simulink model "Robot Michał Krzyszczuk"  (R2018b)
settings: Solver=VariableStepAuto  StartTime=0.0  StopTime=500  MaxStep=0.001  RelTol=1e-3
libraries: commrandsrc3 x9
settings Model: Creator=lenovo  LastModifiedBy=michask
settings SFSimCC: SimUseLocalCustomCode=off
settings RTWCC: RTWUseLocalCustomCode=off
settings CodeAppCC: StateflowObjectComments=on

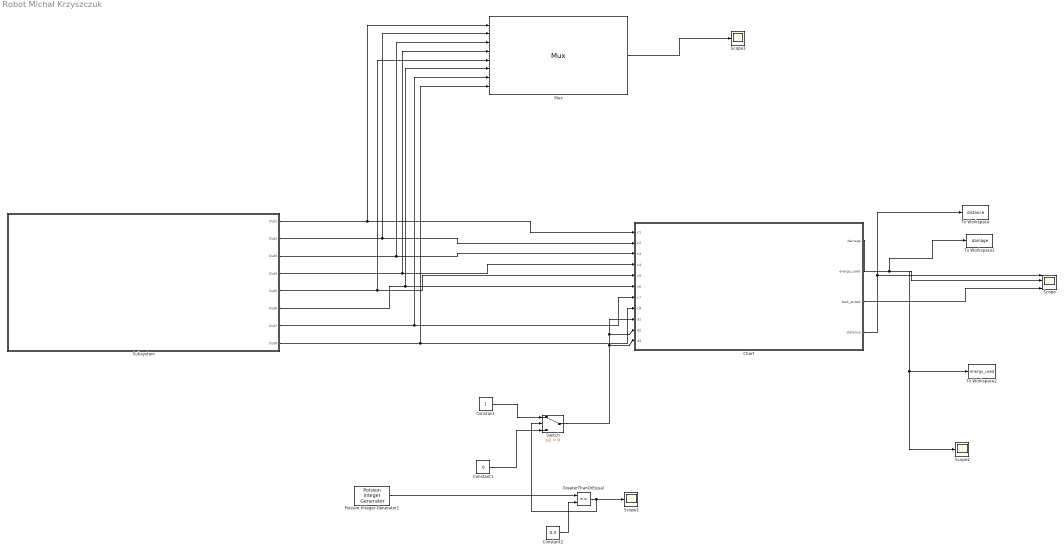
== system Robot Michał Krzyszczuk ==
  Chart : Stateflow chart  TreatAsAtomicUnit=on
  Constant : Constant
  Constant1 : Constant  Value=0
  Constant2 : Constant  Value=0.5
  GreaterThanOrEqual : RelationalOperator  OutDataTypeStr=boolean  RndMeth=Simplest
  Mux : Mux  Inputs=8
  Poisson Integer Generator1 : commrandsrc3/Poisson Integer Generator  PoissonParameter=0.01  SeedSource=Auto  Seed=0  SampleTime=0.1  SamplesPerFrame=1  OutputDataType=double  SimulateUsing=Interpreted execution
      settings: SourceProductName=Communications System Toolbox  SourceProductBaseCode=CM
  Scope : Scope  NumInputPorts=4
  Scope1 : Scope
  Scope2 : Scope
  Scope3 : Scope
  Subsystem : Subsystem
  Switch : Switch  Criteria=u2 > Threshold
  To Workspace : ToWorkspace  VariableName=distance  SampleTime=-1
  To Workspace1 : ToWorkspace  VariableName=damage  SampleTime=-1
  To Workspace2 : ToWorkspace  VariableName=energy_used  SampleTime=-1
  wires:
  Chart/1(damage) -> To Workspace1/1, Scope/2
  Subsystem/1(Out1) -> Mux/1, Chart/1(c1)
  Subsystem/2(Out2) -> Mux/2, Chart/2(c2)
  Subsystem/3(Out3) -> Mux/3, Chart/3(c3)
  Subsystem/4(Out4) -> Mux/4, Chart/4(c4)
  Subsystem/5(Out5) -> Mux/5, Chart/5(c5)
  Subsystem/6(Out6) -> Mux/6, Chart/6(c6)
  Subsystem/7(Out7) -> Mux/7, Chart/7(c7)
  Subsystem/8(Out8) -> Mux/8, Chart/8(c8)
  Constant1/1 -> Switch/3
  Constant/1 -> Switch/1
  Poisson Integer Generator1/1 -> GreaterThanOrEqual/1
  GreaterThanOrEqual/1 -> Scope1/1, Switch/2
  Constant2/1 -> GreaterThanOrEqual/2
  Switch/1 -> Chart/11(d3), Chart/9(d1), Chart/10(d2)
  Chart/2(energy_used) -> Scope2/1, To Workspace2/1
  Chart/3(task_ended) -> Scope/4
  Chart/4(distance) -> Scope/1, To Workspace/1
  Mux/1 -> Scope3/1

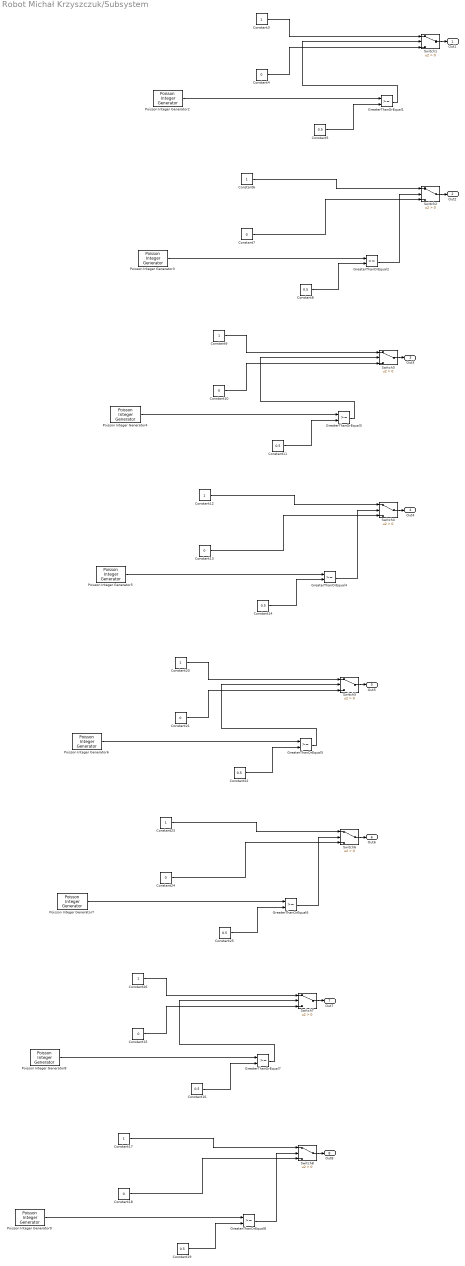
== system Robot Michał Krzyszczuk/Subsystem ==
  Constant{4,7,10,13,15,18,21,24} (8 alike) : Constant  Value=0
  Constant{5,8,11,14,16,19,22,25} (8 alike) : Constant  Value=0.5
  Constant{3,6,9,12,17,20,23,26} (8 alike) : Constant
  GreaterThanOrEqual{1..8} (8 alike) : RelationalOperator  OutDataTypeStr=boolean  RndMeth=Simplest
  Poisson Integer Generator{2..9} (8 alike) : commrandsrc3/Poisson Integer Generator  PoissonParameter=0.08  SeedSource=Auto  Seed=0  SampleTime=0.1  SamplesPerFrame=1  OutputDataType=double  SimulateUsing=Interpreted execution
      settings: SourceProductName=Communications System Toolbox  SourceProductBaseCode=CM
  Switch{1..8} (8 alike) : Switch  Criteria=u2 > Threshold
  Out1 : Outport
  Out2 : Outport  Port=2
  Out3 : Outport  Port=3
  Out4 : Outport  Port=4
  Out5 : Outport  Port=5
  Out6 : Outport  Port=6
  Out7 : Outport  Port=7
  Out8 : Outport  Port=8
  wires:
  GreaterThanOrEqual3/1 -> Switch3/2
  Constant9/1 -> Switch3/1
  Constant25/1 -> GreaterThanOrEqual6/2
  Constant15/1 -> Switch7/3
  Constant10/1 -> Switch3/3
  Constant6/1 -> Switch2/1
  Constant11/1 -> GreaterThanOrEqual3/2
  Switch7/1 -> Out7/1
  Constant13/1 -> Switch4/3
  Switch8/1 -> Out8/1
  Constant24/1 -> Switch6/3
  Constant14/1 -> GreaterThanOrEqual4/2
  Poisson Integer Generator5/1 -> GreaterThanOrEqual4/1
  GreaterThanOrEqual4/1 -> Switch4/2
  Switch5/1 -> Out5/1
  Constant20/1 -> Switch5/1
  Poisson Integer Generator4/1 -> GreaterThanOrEqual3/1
  GreaterThanOrEqual7/1 -> Switch7/2
  Poisson Integer Generator2/1 -> GreaterThanOrEqual1/1
  Constant12/1 -> Switch4/1
  Constant26/1 -> Switch7/1
  Constant7/1 -> Switch2/3
  Constant21/1 -> Switch5/3
  Poisson Integer Generator8/1 -> GreaterThanOrEqual7/1
  Constant19/1 -> GreaterThanOrEqual8/2
  GreaterThanOrEqual1/1 -> Switch1/2
  Constant3/1 -> Switch1/1
  GreaterThanOrEqual5/1 -> Switch5/2
  GreaterThanOrEqual6/1 -> Switch6/2
  Constant22/1 -> GreaterThanOrEqual5/2
  Poisson Integer Generator6/1 -> GreaterThanOrEqual5/1
  Poisson Integer Generator7/1 -> GreaterThanOrEqual6/1
  GreaterThanOrEqual8/1 -> Switch8/2
  Poisson Integer Generator9/1 -> GreaterThanOrEqual8/1
  Constant17/1 -> Switch8/1
  Constant4/1 -> Switch1/3
  Poisson Integer Generator3/1 -> GreaterThanOrEqual2/1
  Constant16/1 -> GreaterThanOrEqual7/2
  Switch6/1 -> Out6/1
  Constant5/1 -> GreaterThanOrEqual1/2
  Switch1/1 -> Out1/1
  Constant23/1 -> Switch6/1
  Constant18/1 -> Switch8/3
  Switch2/1 -> Out2/1
  Constant8/1 -> GreaterThanOrEqual2/2
  GreaterThanOrEqual2/1 -> Switch2/2
  Switch3/1 -> Out3/1
  Switch4/1 -> Out4/1

== stateflow chart Robot Michał Krzyszczuk/Chart ==
  state P
    entry:
    damage_prop=rand;
    p11=rand;
  state H
    entry:
    damage_prop=rand;
    if(damage_prop>0.89) damage=damage-0.004; end;
    p12=rand;
    p3=rand;
  state M
    entry:
    energy_used = energy_used +0.00005;
    p10=rand;
  state Init
    entry: distance=0.06;%moj parametr
    damage=1;
    damage_prop=0;
    r1=0.05;
    r2=0.06;
    r3=0.8;
    r4=0.01;
    r5=0.5;
    r6=0.01;
    r7=1-r5;
    r8=0.01;
    r9=0.01;
    r10=0.01;
    r11=0.02;
    r12 = 1-r3;
  state C
    entry:
    damage_prop=rand;
    energy_used = energy_used+0.00015
    if(damage_prop>0.9895) damage=damage-0.0005; end;
    p9=rand;
  state E
    entry:
    if(distance>6.28) distance=0; end;
    damage_prop=rand;
    energy_used = energy_used+0.0001;
    if(damage_prop>0.9995) damage=damage-0.0021; end;
    p1=rand;
    p2=rand;
    p4=rand;
  state D
    entry:
    damage_prop=rand;
    pd1=rand;
    pd2=rand;
  state F
    en:
    task_ended = 1
  state R
    entry:
    p5=rand;
    p7=rand;
    if damage <=0
    damage = 1
    end
  state W
    entry:
    pd3=rand;
    p8=rand;
  P -> M [order 5] : [c2>0]
  M -> P [order 1] : [c3>0]
  H -> P [order 1] : [p12<=r12]
  M -> R [order 4] : [p10<=r10]
  P -> H [order 2] : [c1>0]
  P -> R [order 4] : [p6<=r6]
  R -> P [order 3] : [p7<=r7]
  M -> E [order 3] : [c5>0]
  M -> F [order 2] : [c7>0]
  E -> M [order 5] : [c4>0]
  E -> P [order 2] : [p1<=r1]
  P -> P [order 3] : after(1,tick)
  P -> E [order 1] : [p11<=r11]
  H -> D [order 2] : [p3<=r3]
  H -> H [order 3] : after(1,tick)
  (default) -> Init
  C -> R [order 1] : [p9<=r9]
  C -> F [order 3] : [c8>0]
  D -> C [order 2] : [d1<=pd1]
  D -> W [order 1] : [d2<=pd2]
  Init -> E
  E -> D [order 1] : [p2<=r2]
  W -> C [order 1] : [d3<=pd3]
  C -> E [order 4] : [c6>0]
  C -> C [order 2] : after(1,tick)
  D -> D [order 3] : after(1,tick)
  E -> E [order 4] : after(1,tick){distance=distance+(2*3.14*0.01)}
  E -> R [order 3] : [p4<=r4]
  R -> E [order 1] : [p5<=r5]
  W -> R [order 2] : [p8<=r6]
  R -> R [order 2] : after(1,tick)
  W -> W [order 3] : after(1,tick)
  data: damage output double; r1 local double; r2 local double; r3 local double; r4 local double; r5 local double; r6 local double; r7 local double; r8 local double; r9 local double; r10 local double; r11 local double; r12 local double; p1 local double; p2 local double; p3 local double; p4 local double; p5 local double; p6 local double =0; p7 local double; p8 local double; p9 local double; p10 local double; p11 local double; p12 local double; pd1 local double =0; pd2 local double =0; pd3 local double =0; c1 input; c2 input; c3 input; c4 input; c5 input; c6 input; c7 input; c8 input; d1 input double; d2 input double; d3 input double; energy_used output =0; task_ended output =0; data local; distance output; damage_prop local
